simulink model "headagent"  (Simulink 6.2)
settings: Solver=ode45  StartTime=0.0  StopTime=10.0  RelTol=1e-3
settings Model: LastModifiedBy=achimk
settings DataIOCC: SignalLoggingName=sigsOut
settings HardwareCC: TargetUnknown=on

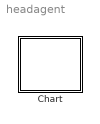
== system headagent ==
  Chart : Stateflow chart

== stateflow chart Chart ==
  state Initialize
    \\Sally\HeadAgent\EyeMotionControl.Initial()
  state MainLoop
    \\Sally\HeadAgent\EyeMotionControl.HeadSample()
    \\Sally\HeadAgent\EyeMotionControl.DoProportionalTracking()
    \\Sally\HeadAgent\EyeMotionControl.WriteMotorPositions()
    \\Sally\HeadAgent\DepthEstimator.FindCartesianCoordinates()
  Initialize -> MainLoop : Always
  MainLoop -> MainLoop : Always
  (default) -> Initialize : Start
